simulink model "Docr_final_UG_spring2022"  (R2020b)
settings: Solver=ode3  StartTime=0.0  StopTime=0.2  FixedStep=1e-6  RelTol=1e-3
InitFcn:
  | Ts=1/1200;
StartFcn:
  | Ts=1/1200;
undefined symbols (not defined in the file): gcbh, sps, sps_rtmsupport
libraries: powerlib x12, powerlib_meascontrol x8, simulink x6
settings Model: Creator=AMLAN SWAIN  LastModifiedBy=Kuldip
settings SolverCC: ZeroCrossAlgorithm=Adaptive
settings DataIOCC: SaveFormat=StructureWithTime  ReturnWorkspaceOutputs=off
settings OptimizationCC: LifeSpan=inf
settings DebuggingCC: IgnoredZcDiagnostic=none  FcnCallInpInsideContextMsg=warning  SFExecutionAtInitializationDiag=none  ArithmeticOperatorsInVariantConditions=warning
settings HardwareCC: ProdBitPerSizeT=32  ProdBitPerPtrDiffT=32  ProdWordSize=32  ProdHWDeviceType=Specified
settings SFSimCC: CustomCodeUndefinedFunction=UseInterfaceOnly
settings CodeAppCC: StateflowObjectComments=on

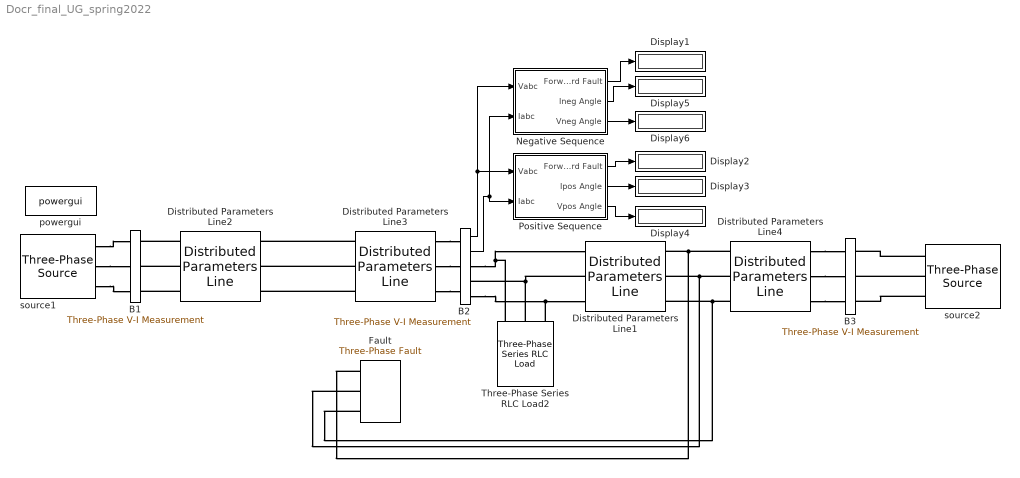
== system Docr_final_UG_spring2022 ==
  B1 : powerlib/Measurements/Three-Phase V-I Measurement  VoltageMeasurement=phase-to-phase  SetLabelV=on  LabelV=Vabc_B1  Vpu=off  VpuLL=off  CurrentMeasurement=yes  SetLabelI=on  LabelI=Iabc_B1  Ipu=off  Pbase=100e6  Vbase=500e3  OutputType=Complex  PhasorSimulation=off  PSBequivalent=0
  B2 : powerlib/Measurements/Three-Phase V-I Measurement  VoltageMeasurement=phase-to-phase  SetLabelV=off  LabelV=Vabc_B2  Vpu=off  VpuLL=off  CurrentMeasurement=yes  SetLabelI=off  LabelI=Iabc_B2  Ipu=off  Pbase=100e6  Vbase=500e3  OutputType=Complex  PhasorSimulation=off  PSBequivalent=0
  B3 : powerlib/Measurements/Three-Phase V-I Measurement  VoltageMeasurement=phase-to-phase  SetLabelV=on  LabelV=Vabc_B4  Vpu=off  VpuLL=off  CurrentMeasurement=yes  SetLabelI=on  LabelI=Iabc_B5  Ipu=off  Pbase=100e6  Vbase=500e3  OutputType=Complex  PhasorSimulation=off  PSBequivalent=0
  Display{1..6} (6 alike) : Display
  Distributed Parameters Line1 : powerlib/Elements/Distributed Parameters Line  Phases=3  Length=0.762  Frequency=60  Resistance=[0.306 0.5919]/1.6  Inductance="[0.6272  2.9855]/(2*3.14*60*1.6)"  Capacitance=[12.74e-9 7.751e-9]  x1=[-5e-06 3.53896556180453e-11 5406.85005261845 -9515.57548770218;-4e-06 3.54057932367556e-11 5410.43695576211 -9513.5364771142;-3e-06 3.54219258235131e-11 5414.02308996202 -9511.49611444051;-2e-06 3.5438053376025e-11 5417.60845470851 -9509.4543999711;-1e-06 3.54541758919991e-11 5421.19304949201 -9507.41133399614]  x2=[-5e-06 -1.85366868295311e-10 5419.21615535197 -9521.95631300143;-4e-06 -1.85400931177469e-10 5422.80546313129 -9519.91264004923;-3e-06 -1.85434967710021e-10 5426.39400020902 -9517.86761410512;-2e-06 -1.85468977888128e-10 5429.98176607514 -9515.82123545977;-1e-06 -1.85502961706956e-10 5433.56876021976 -9513.773504404]  x3=[-5e-06 5.85879936355648e-11 17.9484980501041 -75.1260423753765;-4e-06 5.85240994258584e-11 17.9768186247305 -75.1192706126395;-3e-06 5.84601968985723e-11 18.0051366444501 -75.1124881737789;-2e-06 5.83962860627885e-11 18.0334521052382 -75.1056950597585;-1e-06 5.83323669275901e-11 18.0617650030706 -75.098891271544]  x4=[-5e-06 -6.22615922122158e-11 19.8872316981426 8.51123101194737;-4e-06 -6.21996822313571e-11 19.8840216265108 8.51872771667214;-3e-06 -6.21377634105364e-11 19.880808728916 8.52622321069571;-2e-06 -6.20758357585537e-11 19.877593005815 8.53371749295282;-1e-06 -6.20138992842104e-11 19.8743744576646 8.54121056237835]  x5=4.72092324098614e-06  V1=[9.374e-10 1.076e+04 1.076e+04;377 377 377;-1.988 0.4876 -1.083]  V2=[8.927e-10 1.062e+04 1.062e+04;377 377 377;-2.049 0.4776 -1.093]  I1=[5.305e-11 493.3 493.3;377 377 377;0.5859 3.134 1.563]  I2=[5.319e-11 560.4 560.4;377 377 377;-2.484 0.05536 -1.515]  nHarmo=1  Measurements=None  Decoupling=off  VsMag0=0  VrMag0=0  VsAngle0=0  VrAngle0=0  IsMag0=0  IrMag0=0  IsAngle0=0  IrAngle0=0
  Distributed Parameters Line2 : powerlib/Elements/Distributed Parameters Line  Phases=3  Length=0.609  Frequency=60  Resistance=[0.306 0.5919]/1.6  Inductance="[0.6272  2.9855]/(2*3.14*60*1.6)"  Capacitance=[12.74e-9 7.751e-9]  x1=[-4e-06 8.87549904824792e-13 0 0;-3e-06 8.93036295222102e-13 5435.11708326214 -9522.75907286486;-2e-06 8.98522558699039e-13 5438.70669254485 -9520.70940534715;-1e-06 9.04008694475882e-13 5442.29552886605 -9518.65838472431]  x2=[-4e-06 -1.48296155558528e-10 0 0;-3e-06 -1.48284057376127e-10 5424.57036035998 -9517.13184208474;-2e-06 -1.48271938119254e-10 5428.15784897618 -9515.08615098768;-1e-06 -1.48259797789633e-10 5431.7445661301 -9513.03910758467]  x3=[-4e-06 -3.76125984754746e-11 0 0;-3e-06 -3.76601196647817e-11 20.6377713668851 11.6240614618364;-2e-06 -3.77076355017458e-11 20.6333877325137 11.6318408921425;-1e-06 -3.7755145979614e-11 20.6290011656777 11.6396186693046]  x4=[-4e-06 3.81367478851825e-11 0 0;-3e-06 3.81846637161445e-11 17.3254740266849 -78.2483135130661;-2e-06 3.82325741202141e-11 17.3549717140448 -78.241776402975;-1e-06 3.82804790905823e-11 17.3844669348762 -78.2352281729825]  x5=3.77302133039443e-06  V1=[4.602e-11 2.2e+05 2.2e+05;377 377 377;2.818 0.5227 -1.048]  V2=[6.708e-11 2.2e+05 2.2e+05;377 377 377;-2.434 0.5227 -1.048]  I1=[6.93e-11 746.2 746.2;377 377 377;-1.328 0.539 -1.032]  I2=[7.511e-11 793.2 793.2;377 377 377;0.4622 0.5065 -1.064]  nHarmo=1  Measurements=None  Decoupling=off  VsMag0=0  VrMag0=0  VsAngle0=0  VrAngle0=0  IsMag0=0  IrMag0=0  IsAngle0=0  IrAngle0=0
  Distributed Parameters Line3 : powerlib/Elements/Distributed Parameters Line  Phases=3  Length=0.609  Frequency=60  Resistance=[0.306 0.5919]/1.6  Inductance="[0.6272  2.9855]/(2*3.14*60*1.6)"  Capacitance=[12.74e-9 7.751e-9]  x1=[-4e-06 -1.79238141052749e-10 0 0;-3e-06 -1.79221258056481e-10 5424.57036036002 -9517.13184208476;-2e-06 -1.79204349588875e-10 5428.15784897622 -9515.0861509877;-1e-06 -1.79187415652335e-10 5431.74456613013 -9513.03910758469]  x2=[-4e-06 1.72104339420921e-11 0 0;-3e-06 1.72279289651859e-11 5414.023089962 -9511.49611444052;-2e-06 1.72454215398067e-11 5417.60845470849 -9509.45439997111;-1e-06 1.72629116634685e-11 5421.19304949199 -9507.41133399616]  x3=[-4e-06 3.22950351945824e-11 0 0;-3e-06 3.23591813475878e-11 20.6287147973381 11.6596262987454;-2e-06 3.24233229016319e-11 20.6243177559832 11.667402312278;-1e-06 3.24874598475987e-11 20.6199177834529 11.6751766676124]  x4=[-4e-06 -2.86355994927887e-11 0 0;-3e-06 -2.86965787344052e-11 17.2607527038474 -78.2444456351624;-2e-06 -2.87575538975978e-11 17.2902489376506 -78.2379329247094;-1e-06 -2.88185249737007e-11 17.3197427141239 -78.2314090949013]  x5=3.77302133039443e-06  V1=[4.602e-11 2.2e+05 2.2e+05;377 377 377;2.818 0.5227 -1.048]  V2=[6.708e-11 2.2e+05 2.2e+05;377 377 377;-2.434 0.5227 -1.048]  I1=[6.93e-11 746.2 746.2;377 377 377;-1.328 0.539 -1.032]  I2=[7.511e-11 793.2 793.2;377 377 377;0.4622 0.5065 -1.064]  nHarmo=1  Measurements=None  Decoupling=off  VsMag0=0  VrMag0=0  VsAngle0=0  VrAngle0=0  IsMag0=0  IrMag0=0  IsAngle0=0  IrAngle0=0
  Distributed Parameters Line4 : powerlib/Elements/Distributed Parameters Line  Phases=3  Length=0.762  Frequency=60  Resistance=[0.306 0.5919]/1.6  Inductance="[0.6272  2.9855]/(2*3.14*60*1.6)"  Capacitance=[12.74e-9 7.751e-9]  x1=[-5e-06 -1.85366868295311e-10 5419.21615535197 -9521.95631300143;-4e-06 -1.85400931177469e-10 5422.80546313129 -9519.91264004923;-3e-06 -1.85434967710021e-10 5426.39400020902 -9517.86761410512;-2e-06 -1.85468977888128e-10 5429.98176607514 -9515.82123545977;-1e-06 -1.85502961706956e-10 5433.56876021976 -9513.773504404]  x2=[-5e-06 -1.83698691120363e-12 5431.58504481057 -9528.32360145216;-4e-06 -1.8333879297796e-12 5435.17675212208 -9526.27526508613;-3e-06 -1.82978868779026e-12 5438.76768697376 -9524.22557482393;-2e-06 -1.82618918574713e-12 5442.35784885526 -9522.17453095687;-1e-06 -1.8225894241618e-12 5445.94723725634 -9520.12213377645]  x3=[-5e-06 -4.22572650147398e-11 18.032001384415 -75.1380771235504;-4e-06 -4.22072207949267e-11 18.060326490101 -75.1312738799439;-3e-06 -4.21571705765263e-11 18.0886490290118 -75.1244599585078;-2e-06 -4.21071143666517e-11 18.1169689971222 -75.1176353602105;-1e-06 -4.20570521724171e-11 18.1452863904072 -75.110800086022]  x4=[-5e-06 3.9105414017705e-11 19.8902302790728 8.47862645586489;-4e-06 3.9054177984932e-11 19.8870324988554 8.48612429334521;-3e-06 3.90029364016894e-11 19.8838318922471 8.493620924758;-2e-06 3.89516892752596e-11 19.8806284597028 8.50111634903784;-1e-06 3.89004366129261e-11 19.8774222016778 8.50861056511946]  x5=4.72092324098614e-06  V1=[9.374e-10 1.076e+04 1.076e+04;377 377 377;-1.988 0.4876 -1.083]  V2=[8.927e-10 1.062e+04 1.062e+04;377 377 377;-2.049 0.4776 -1.093]  I1=[5.305e-11 493.3 493.3;377 377 377;0.5859 3.134 1.563]  I2=[5.319e-11 560.4 560.4;377 377 377;-2.484 0.05536 -1.515]  nHarmo=1  Measurements=None  Decoupling=off  VsMag0=0  VrMag0=0  VsAngle0=0  VrAngle0=0  IsMag0=0  IrMag0=0  IsAngle0=0  IrAngle0=0
  Fault : powerlib/Elements/Three-Phase Fault  InitialStates=0  FaultA=on  FaultB=off  FaultC=off  GroundFault=on  SwitchTimes=[0.1]  External=off  SwitchStatus=NaN  FaultResistance=2  GroundResistance=0.01  SnubberResistance=1e6  SnubberCapacitance=inf  Measurements=None
  Negative Sequence : Subsystem
  Positive Sequence : Subsystem
  Three-Phase Series RLC Load2 : powerlib/Elements/Three-Phase Series RLC Load  LConnTagsString=A|B|C  Configuration=Y (grounded)  NominalVoltage=11e3  Vabc=[1e3 1e3 1e3]  Vabcp=[1e3 1e3 1e3]  NominalFrequency=60  UnbalancedPower=off  ActivePower=0.82e6  InductivePower=0.5e6  CapacitivePower=0  Pabc=[10e3 9e3 11e3]  QLabc=[100 90 110]  QCabc=[100 90 110]  Pabcp=[10e3 9e3 11e3]  QLabcp=[100 90 110]  QCabcp=[100 90 110]  Measurements=None  LoadType=constant Z
  powergui : powerlib/powergui  Priority=1  SimulationMode=Discrete  SampleTime=1e-6  frequency=60  Iterations=50  frequencyindice=0  Pbase=100e6  ErrMax=1e-4  UnitsV=kV  UnitsW=MW  buscounter=0  FunctionMessages=off  echomessages=off  EnableUseOfTLC=off  CurrentSourceSwitches=off  DisableSnubberDevices=off  DisableRonSwitches=off  DisableVfSwitches=off  DisplayEquations=off  AutomaticDiscreteSolvers=off  SolverType=Tustin/Backward Euler (TBE)  Interpol=off  ExternalGateDelay=off  methode=off  Ts=100  x0status=blocks  SPID=off  SwTol=0  HookPort=off  NonlinearTolerance=1e-4  nMaxIteration=100  ContinueOnMaxIteration=off  RestoreLinks=warning  ResistiveCurrentMeasurement=off  Frange=[0:2:500]  Ylog=off  Xlog=on  ShowGrid=off  save=off  variable=ZData  structure=dcneg  ZoomFFT=off  StartTime=0.1  cycles=3  DisplayStyle=1  fundamental=60  FreqAxis=off  MaxFrequency=1000  frequencyindicesteady=1  RmsSteady=1  display=off
  source1 : powerlib/Electrical Sources/Three-Phase Source  InternalConnection=Yg  VoltagePhases=off  Voltage=11e3  PhaseAngle=0  Voltage_phases=[220e3 220e3 220e3]/sqrt(3)  PhaseAngles_phases=[0]  Frequency=60  NonIdealSource=on  SpecifyImpedance=on  Resistance=0.8929  Inductance=0.025  ShortCircuitLevel=100e6  BaseVoltage=11e3  XRratio=7  BusType=swing  Pref=10e3  Qref=0  Prefabc=[10e3, 10e3, 10e3]  Qrefabc=[0, 0, 0]  Qmin=-inf  Qmax=inf
  source2 : powerlib/Electrical Sources/Three-Phase Source  InternalConnection=Yg  VoltagePhases=off  Voltage=11e3  PhaseAngle=0  Voltage_phases=[220e3 220e3 220e3]/sqrt(3)  PhaseAngles_phases=[0]  Frequency=60  NonIdealSource=on  SpecifyImpedance=on  Resistance=0.8929  Inductance=0.025  ShortCircuitLevel=100e6  BaseVoltage=11e3  XRratio=7  BusType=swing  Pref=10e3  Qref=0  Prefabc=[10e3, 10e3, 10e3]  Qrefabc=[0, 0, 0]  Qmin=-inf  Qmax=inf
  wires:
  Positive Sequence/1(Forward Fault) -> Display2/1
  B2/1 -> Negative Sequence/1(Vabc), Positive Sequence/1(Vabc)
  B2/2 -> Negative Sequence/2(Iabc), Positive Sequence/2(Iabc)
  Negative Sequence/1(Forward Fault) -> Display1/1
  Positive Sequence/2(Ipos Angle) -> Display3/1
  Positive Sequence/3(Vpos Angle) -> Display4/1
  Negative Sequence/2(Ineg Angle) -> Display5/1
  Negative Sequence/3(Vneg Angle) -> Display6/1
  connections:
  source2/RConn1 -- B3/LConn1
  source2/RConn2 -- B3/LConn2
  source2/RConn3 -- B3/LConn3
  Distributed Parameters Line2/LConn1 -- B1/RConn1
  Distributed Parameters Line2/LConn2 -- B1/RConn2
  Distributed Parameters Line2/LConn3 -- B1/RConn3
  Distributed Parameters Line1/LConn2 -- B2/RConn2 -- Three-Phase Series RLC Load2/LConn2
  B2/RConn1 -- Three-Phase Series RLC Load2/LConn1 -- Distributed Parameters Line1/LConn1
  B2/RConn3 -- Three-Phase Series RLC Load2/LConn3 -- Distributed Parameters Line1/LConn3
  source1/RConn2 -- B1/LConn2
  source1/RConn1 -- B1/LConn1
  source1/RConn3 -- B1/LConn3
  Distributed Parameters Line3/LConn1 -- Distributed Parameters Line2/RConn1
  Distributed Parameters Line3/LConn2 -- Distributed Parameters Line2/RConn2
  Distributed Parameters Line3/LConn3 -- Distributed Parameters Line2/RConn3
  Distributed Parameters Line3/RConn1 -- B2/LConn1
  Distributed Parameters Line3/RConn2 -- B2/LConn2
  Distributed Parameters Line3/RConn3 -- B2/LConn3
  Distributed Parameters Line4/LConn1 -- Fault/LConn1 -- Distributed Parameters Line1/RConn1
  Distributed Parameters Line4/LConn2 -- Fault/LConn2 -- Distributed Parameters Line1/RConn2
  Distributed Parameters Line4/LConn3 -- Fault/LConn3 -- Distributed Parameters Line1/RConn3
  Distributed Parameters Line4/RConn1 -- B3/RConn1
  Distributed Parameters Line4/RConn2 -- B3/RConn2
  Distributed Parameters Line4/RConn3 -- B3/RConn3

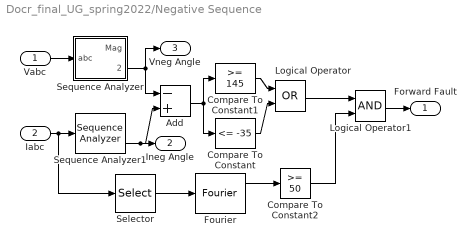
== system Docr_final_UG_spring2022/Negative Sequence ==
  Vabc : Inport
  Iabc : Inport  Port=2
  Add : Sum  Inputs=-+
  Compare To Constant : simulink/Logic and Bit Operations/Compare To Constant  relop=<=  const=-35  OutDataTypeStr=boolean
  Compare To Constant1 : simulink/Logic and Bit Operations/Compare To Constant  relop=>=  const=145  OutDataTypeStr=boolean
  Compare To Constant2 : simulink/Logic and Bit Operations/Compare To Constant  relop=>=  const=50  OutDataTypeStr=boolean
  Fourier : powerlib_meascontrol/Measurements/Fourier  Freq=60  n=1  InInit=[0, 0]  Ts=0
  Logical Operator : Logic  Operator=OR  AllPortsSameDT=off  OutDataTypeStr=boolean
  Logical Operator1 : Logic  AllPortsSameDT=off  OutDataTypeStr=boolean
  Selector : Selector  InputPortWidth=3  IndexOptions=Index vector (dialog)  Indices=[1 ]  OutputSizes=1
  Sequence Analyzer : Subsystem  AncestorBlock=powerlib_meascontrol/Measurements/Sequence Analyzer  DialogController=POWERSYS.PowerSysDialog  LoadFcn=sps_rtmsupport('LoadFcn', gcbh);  StartFcn=sps_rtmsupport('StartFcn', gcbh);  StopFcn=sps_rtmsupport('StopFcn', gcbh);  mask(Sequence Analyzer){Freq=60, n=1, seq=Negative, InInit=[1, 0], Ts=0}
      mask prompts: Freq "Fundamental frequency (Hz):"; n "Harmonic n (1=fundamental):"; seq "Sequence:"; InInit "Initial input [ Mag, Phase (degrees) ]:"; Ts "Sample time:"
      mask help: Compute the positive-, negative-, and zero-sequence components of a three-phase signal.
      mask init:
      | [WantBlockChoice,Ts,sps] = powericon('SequenceAnalyzerInit',gcb,Freq,n,seq,InInit,Ts);
      settings: CopyFcn=sps_rtmsupport('CopyFcn', gcbh);  DeleteFcn=sps_rtmsupport('DeleteFcn', gcbh);  UndoDeleteFcn=sps_rtmsupport('UndoDeleteFcn', gcbh);  ModelCloseFcn=sps_rtmsupport('ModelCloseFcn', gcbh);  PreSaveFcn=sps_rtmsupport('PreSaveFcn', gcbh);  PostSaveFcn=sps_rtmsupport('PostSaveFcn', gcbh);  NameChangeFcn=sps_rtmsupport('NameChangeFcn', gcbh);  PreCopyFcn=sps_rtmsupport('PreCopyFcn', gcbh);  OpenFcn=sps_rtmsupport('OpenFcn', gcbh, [3]);  CloseFcn=sps_rtmsupport('CloseFcn', gcbh);  PreDeleteFcn=sps_rtmsupport('PreDeleteFcn', gcbh);
      mask Help: helpview(psbhelp);
      mask TypeOptions seq: Positive | Negative | Zero | Positive Negative Zero
      mask Display:
      | port_label('input',1,'abc')
      | port_label('output',1,'|u|')
      | port_label('output',2,'\angleu', 'texmode', 'on')
  Sequence Analyzer1 : powerlib_meascontrol/Measurements/Sequence Analyzer  Freq=60  n=1  seq=Negative  InInit=[1, 0]  Ts=0
      settings: SourceProductBaseCode=PS
  Forward Fault : Outport
  Ineg Angle : Outport  Port=2
  Vneg Angle : Outport  Port=3
  wires:
  Sequence Analyzer1/2 -> Add/2, Ineg Angle/1
  Vabc/1 -> Sequence Analyzer/1(abc)
  Add/1 -> Compare To Constant/1, Compare To Constant1/1
  Compare To Constant1/1 -> Logical Operator/1
  Compare To Constant/1 -> Logical Operator/2
  Sequence Analyzer/2(Phase(-)) -> Vneg Angle/1, Add/1
  Fourier/1 -> Compare To Constant2/1
  Selector/1 -> Fourier/1
  Compare To Constant2/1 -> Logical Operator1/2
  Iabc/1 -> Selector/1, Sequence Analyzer1/1
  Logical Operator/1 -> Logical Operator1/1
  Logical Operator1/1 -> Forward Fault/1

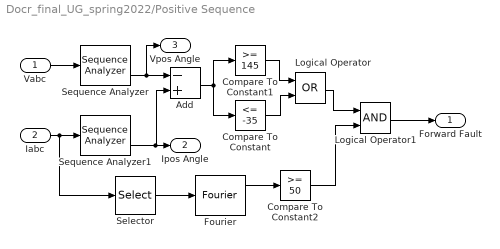
== system Docr_final_UG_spring2022/Positive Sequence ==
  Vabc : Inport
  Iabc : Inport  Port=2
  Add : Sum  Inputs=-+
  Compare To Constant : simulink/Logic and Bit Operations/Compare To Constant  relop=<=  const=-35  OutDataTypeStr=boolean
  Compare To Constant1 : simulink/Logic and Bit Operations/Compare To Constant  relop=>=  const=145  OutDataTypeStr=boolean
  Compare To Constant2 : simulink/Logic and Bit Operations/Compare To Constant  relop=>=  const=50  OutDataTypeStr=boolean
  Fourier : powerlib_meascontrol/Measurements/Fourier  Freq=60  n=1  InInit=[0, 0]  Ts=0
  Logical Operator : Logic  Operator=OR  AllPortsSameDT=off  OutDataTypeStr=boolean
  Logical Operator1 : Logic  AllPortsSameDT=off  OutDataTypeStr=boolean
  Selector : Selector  InputPortWidth=3  IndexOptions=Index vector (dialog)  Indices=[1 ]  OutputSizes=1
  Sequence Analyzer : powerlib_meascontrol/Measurements/Sequence Analyzer  Freq=60  n=1  seq=Positive  InInit=[1, 0]  Ts=0
      settings: SourceProductBaseCode=PS
  Sequence Analyzer1 : powerlib_meascontrol/Measurements/Sequence Analyzer  Freq=60  n=1  seq=Positive  InInit=[1, 0]  Ts=0
      settings: SourceProductBaseCode=PS
  Forward Fault : Outport
  Ipos Angle : Outport  Port=2
  Vpos Angle : Outport  Port=3
  wires:
  Sequence Analyzer1/2 -> Ipos Angle/1, Add/2
  Sequence Analyzer/2 -> Vpos Angle/1, Add/1
  Vabc/1 -> Sequence Analyzer/1
  Iabc/1 -> Selector/1, Sequence Analyzer1/1
  Add/1 -> Compare To Constant/1, Compare To Constant1/1
  Logical Operator/1 -> Logical Operator1/1
  Compare To Constant1/1 -> Logical Operator/1
  Compare To Constant/1 -> Logical Operator/2
  Selector/1 -> Fourier/1
  Fourier/1 -> Compare To Constant2/1
  Compare To Constant2/1 -> Logical Operator1/2
  Logical Operator1/1 -> Forward Fault/1

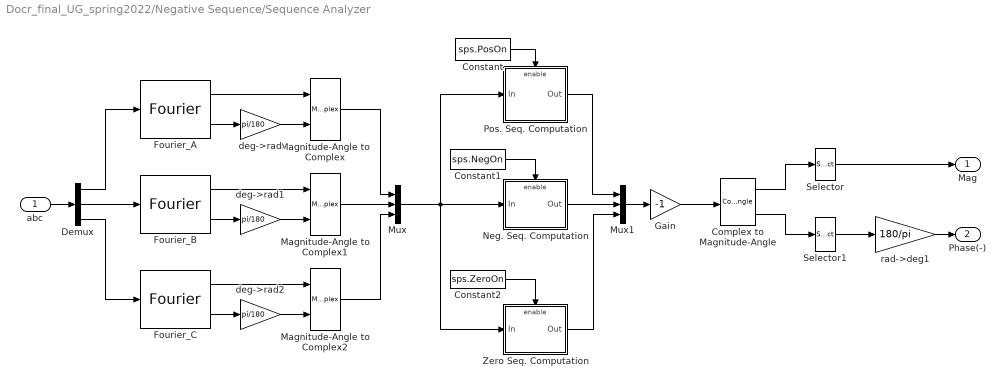
== system Docr_final_UG_spring2022/Negative Sequence/Sequence Analyzer ==
  abc : Inport  PortDimensions=3  SampleTime=Ts
  Complex to Magnitude-Angle : ComplexToMagnitudeAngle
  Constant : Constant  Value=sps.PosOn
  Constant1 : Constant  Value=sps.NegOn
  Constant2 : Constant  Value=sps.ZeroOn
  Demux : Demux  Outputs=3
  Fourier_A : powerlib_meascontrol/Measurements/Fourier  Freq=sps.Freq  n=sps.n  InInit=sps.Par_Init  Ts=Ts
  Fourier_B : powerlib_meascontrol/Measurements/Fourier  Freq=sps.Freq  n=sps.n  InInit="[sps.Par_Init(1)  sps.Par_Init(2)-120 ]"  Ts=Ts
  Fourier_C : powerlib_meascontrol/Measurements/Fourier  Freq=sps.Freq  n=sps.n  InInit="[sps.Par_Init(1)  sps.Par_Init(2)+120 ]"  Ts=Ts
  Gain : Gain  Gain=-1
  Magnitude-Angle to Complex : MagnitudeAngleToComplex
  Magnitude-Angle to Complex1 : MagnitudeAngleToComplex
  Magnitude-Angle to Complex2 : MagnitudeAngleToComplex
  Mux : Mux  Inputs=3
  Mux1 : Mux  Inputs=3
  Neg. Seq. Computation : Subsystem  TreatAsAtomicUnit=on
  Pos. Seq. Computation : Subsystem  TreatAsAtomicUnit=on
  Selector : Selector  InputPortWidth=3  IndexOptions=Index vector (dialog)  Indices=sps.SelectElement  OutputSizes=1
  Selector1 : Selector  InputPortWidth=3  IndexOptions=Index vector (dialog)  Indices=sps.SelectElement  OutputSizes=1
  Zero Seq. Computation : Subsystem  TreatAsAtomicUnit=on
  deg->rad : Gain  Gain=pi/180  SaturateOnIntegerOverflow=on  OutDataTypeStr=Inherit: Same as input  ParamDataTypeStr=Inherit: Same as input
  deg->rad1 : Gain  Gain=pi/180  SaturateOnIntegerOverflow=on  OutDataTypeStr=Inherit: Same as input  ParamDataTypeStr=Inherit: Same as input
  deg->rad2 : Gain  Gain=pi/180  SaturateOnIntegerOverflow=on  OutDataTypeStr=Inherit: Same as input  ParamDataTypeStr=Inherit: Same as input
  rad->deg1 : Gain  Gain=180/pi  SaturateOnIntegerOverflow=on  OutDataTypeStr=Inherit: Same as input  ParamDataTypeStr=Inherit: Same as input
  Mag : Outport  SampleTime=Ts  InitialOutput=0
  Phase(-) : Outport  Port=2  SampleTime=Ts  InitialOutput=0
  wires:
  Selector1/1 -> rad->deg1/1
  Magnitude-Angle to Complex2/1 -> Mux/3
  Magnitude-Angle to Complex1/1 -> Mux/2
  Magnitude-Angle to Complex/1 -> Mux/1
  Fourier_C/2 -> deg->rad2/1
  deg->rad2/1 -> Magnitude-Angle to Complex2/2
  Fourier_C/1 -> Magnitude-Angle to Complex2/1
  Fourier_B/2 -> deg->rad1/1
  deg->rad1/1 -> Magnitude-Angle to Complex1/2
  Fourier_B/1 -> Magnitude-Angle to Complex1/1
  deg->rad/1 -> Magnitude-Angle to Complex/2
  Fourier_A/2 -> deg->rad/1
  Fourier_A/1 -> Magnitude-Angle to Complex/1
  Demux/3 -> Fourier_C/1
  Demux/2 -> Fourier_B/1
  Demux/1 -> Fourier_A/1
  abc/1 -> Demux/1
  Constant1/1 -> Neg. Seq. Computation/Enable
  Complex to Magnitude-Angle/2 -> Selector1/1
  Selector/1 -> Mag/1
  Constant2/1 -> Zero Seq. Computation/Enable
  Constant/1 -> Pos. Seq. Computation/Enable
  Complex to Magnitude-Angle/1 -> Selector/1
  Zero Seq. Computation/1(Out) -> Mux1/3
  Neg. Seq. Computation/1(Out) -> Mux1/2
  Pos. Seq. Computation/1(Out) -> Mux1/1
  Mux/1 -> Zero Seq. Computation/1(In), Neg. Seq. Computation/1(In), Pos. Seq. Computation/1(In)
  Gain/1 -> Complex to Magnitude-Angle/1
  Mux1/1 -> Gain/1
  rad->deg1/1 -> Phase(-)/1

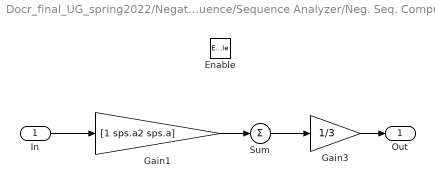
== system Docr_final_UG_spring2022/Negative Sequence/Sequence Analyzer/Neg. Seq. Computation ==
  In : Inport
  Enable : EnablePort  PropagateVarSize=During execution
  Gain1 : Gain  Gain=[1 sps.a2 sps.a]  SaturateOnIntegerOverflow=on  OutDataTypeStr=Inherit: Same as input  ParamDataTypeStr=Inherit: Same as input
  Gain3 : Gain  Gain=1/3  SaturateOnIntegerOverflow=on  OutDataTypeStr=Inherit: Same as input  ParamDataTypeStr=Inherit: Same as input
  Sum : Sum  Inputs=1  InputSameDT=on  SaturateOnIntegerOverflow=on  OutDataTypeStr=Inherit: Same as first input
  Out : Outport
  wires:
  Gain3/1 -> Out/1
  In/1 -> Gain1/1
  Sum/1 -> Gain3/1
  Gain1/1 -> Sum/1

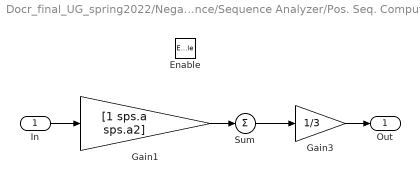
== system Docr_final_UG_spring2022/Negative Sequence/Sequence Analyzer/Pos. Seq. Computation ==
  In : Inport
  Enable : EnablePort  PropagateVarSize=During execution
  Gain1 : Gain  Gain=[1 sps.a sps.a2]  SaturateOnIntegerOverflow=on  OutDataTypeStr=Inherit: Same as input  ParamDataTypeStr=Inherit: Same as input
  Gain3 : Gain  Gain=1/3  SaturateOnIntegerOverflow=on  OutDataTypeStr=Inherit: Same as input  ParamDataTypeStr=Inherit: Same as input
  Sum : Sum  Inputs=1  InputSameDT=on  SaturateOnIntegerOverflow=on  OutDataTypeStr=Inherit: Same as first input
  Out : Outport
  wires:
  Gain3/1 -> Out/1
  In/1 -> Gain1/1
  Sum/1 -> Gain3/1
  Gain1/1 -> Sum/1

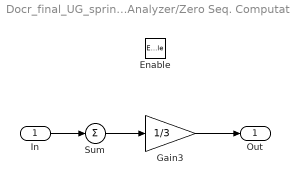
== system Docr_final_UG_spring2022/Negative Sequence/Sequence Analyzer/Zero Seq. Computation ==
  In : Inport
  Enable : EnablePort  PropagateVarSize=During execution
  Gain3 : Gain  Gain=1/3  SaturateOnIntegerOverflow=on  OutDataTypeStr=Inherit: Same as input  ParamDataTypeStr=Inherit: Same as input
  Sum : Sum  Inputs=1  InputSameDT=on  SaturateOnIntegerOverflow=on  OutDataTypeStr=Inherit: Same as first input
  Out : Outport
  wires:
  Gain3/1 -> Out/1
  In/1 -> Sum/1
  Sum/1 -> Gain3/1
